simulink library "Library"  (R2020b)
settings: Solver=VariableStepAuto  StartTime=0.0  StopTime=10.0  RelTol=1e-3
settings Model: Creator=mulusoy  LastModifiedBy=keati
settings DataIOCC: ReturnWorkspaceOutputs=off
settings DebuggingCC: ArithmeticOperatorsInVariantConditions=warning
settings SFSimCC: SimUseLocalCustomCode=off  CustomCodeUndefinedFunction=UseInterfaceOnly
settings RTWCC: RTWUseLocalCustomCode=off

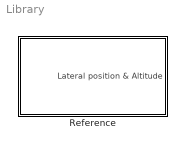
== system Library ==
  Reference : Subsystem
      mask Display: image("Reference.jpg");

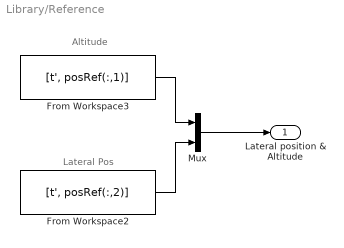
== system Library/Reference ==
  note: Lateral Pos
  note: Altitude
  From Workspace2 : FromWorkspace  VariableName=[t', posRef(:,2)]  SampleTime=.1
  From Workspace3 : FromWorkspace  VariableName=[t', posRef(:,1)]  SampleTime=.1
  Mux : Mux  Inputs=2
  Lateral position & Altitude : Outport  VectorParamsAs1DForOutWhenUnconnected=off
  wires:
  Mux/1 -> Lateral position & Altitude/1
  From Workspace2/1 -> Mux/2
  From Workspace3/1 -> Mux/1
